simulink model "Quanser_AERO_Simulation_2020b"  (R2020b)
settings: Solver=ode45  StartTime=0.0  StopTime=sim_time  FixedStep=0.01  RelTol=1e-3
InitFcn:
  | % Run simulation parameters
  | quanser_AERO_sim_params;
model workspace (MAT data in the model file):
  a = Simulink.Parameter
  a.Value = 1.15
  a.DataType = 'auto'
  a.Dimensions = [1 1]
  a_a = Simulink.Parameter
  a_a.Value = 0.043381
  a_a.DataType = 'auto'
  a_a.Dimensions = [1 1]
  b = Simulink.Parameter
  b.Value = 0.2847
  b.DataType = 'auto'
  b.Dimensions = [1 1]
  b_b = Simulink.Parameter
  b_b.Value = 0.005
  b_b.DataType = 'auto'
  b_b.Dimensions = [1 1]
  c = Simulink.Parameter
  c.Value = 0.53573
  c.DataType = 'auto'
  c.Dimensions = [1 1]
  c_c = Simulink.Parameter
  c_c.Value = 0.005
  c_c.DataType = 'auto'
  c_c.Dimensions = [1 1]
  d = Simulink.Parameter
  d.Value = 0.0071058
  d.DataType = 'auto'
  d.Dimensions = [1 1]
  d_d = Simulink.Parameter
  d_d.Value = 0
  d_d.DataType = 'auto'
  d_d.Dimensions = [1 1]
  e = Simulink.Parameter
  e.Value = 0.0071
  e.DataType = 'auto'
  e.Dimensions = [1 1]
  f = Simulink.Parameter
  f.Value = 0.05
  f.DataType = 'auto'
  f.Dimensions = [1 1]
  g = Simulink.Parameter
  g.Value = 9.81
  g.DataType = 'auto'
  g.Dimensions = [1 1]
  p_p = Simulink.Parameter
  p_p.Value = 0.0005466
  p_p.DataType = 'auto'
  p_p.Dimensions = [1 1]
  smiData.RigidTransform(1).translation = [75 240 -4.4408920985e-15]
  smiData.RigidTransform(1).angle = 1.57079632679
  smiData.RigidTransform(1).axis = [5.55111512313e-17 1 5.55111512313e-17]
  smiData.RigidTransform(1).ID = 'B[AERO - Fork:1:-:AERO - Arm:1]'
  smiData.RigidTransform(2).translation = [0 0 72.5]
  smiData.RigidTransform(2).angle = 0
  smiData.RigidTransform(2).axis = [0 0 0]
  smiData.RigidTransform(2).ID = 'F[AERO - Fork:1:-:AERO - Arm:1]'
  smiData.RigidTransform(3).translation = [53 0 0]
  smiData.RigidTransform(3).angle = 1.57079632679
  smiData.RigidTransform(3).axis = [0 -1 0]
  smiData.RigidTransform(3).ID = 'B[AERO - Arm:1:-:AERO - Propeller Housing:1]'
  smiData.RigidTransform(4).translation = [-2.67952073108e-14 10 -95.5137103749]
  smiData.RigidTransform(4).angle = 3.14159265359
  smiData.RigidTransform(4).axis = [1 0 0]
  smiData.RigidTransform(4).ID = 'F[AERO - Arm:1:-:AERO - Propeller Housing:1]'
  smiData.RigidTransform(5).translation = [-53 0 0]
  smiData.RigidTransform(5).angle = 3.14159265359
  smiData.RigidTransform(5).axis = [0.707106781187 0 0.707106781187]
  smiData.RigidTransform(5).ID = 'B[AERO - Arm:1:-:AERO - Propeller Housing:2]'
  smiData.RigidTransform(6).translation = [-2.67952073108e-14 10 -95.5137103749]
  smiData.RigidTransform(6).angle = 3.14159265359
  smiData.RigidTransform(6).axis = [1 0 0]
  smiData.RigidTransform(6).ID = 'F[AERO - Arm:1:-:AERO - Propeller Housing:2]'
  smiData.RigidTransform(7).translation = [0 90 0]
  smiData.RigidTransform(7).angle = 2.09439510239
  smiData.RigidTransform(7).axis = [-0.57735026919 -0.57735026919 -0.57735026919]
  smiData.RigidTransform(7).ID = 'B[AERO - Base:1:-:AERO - Fork:1]'
  smiData.RigidTransform(8).translation = [0 -10 -1.83697019872e-15]
  smiData.RigidTransform(8).angle = 1.57079632679
  smiData.RigidTransform(8).axis = [-1 0 0]
  smiData.RigidTransform(8).ID = 'F[AERO - Base:1:-:AERO - Fork:1]'
  smiData.RigidTransform(9).translation = [0 7 0]
  smiData.RigidTransform(9).angle = 1.57079632679
  smiData.RigidTransform(9).axis = [-1 1.5327705937e-16 1.5327705937e-16]
  smiData.RigidTransform(9).ID = 'B[AERO - Propeller Housing:1:-:AERO - Propeller:1]'
  smiData.RigidTransform(10).translation = [0 2 0]
  smiData.RigidTransform(10).angle = 1.6664335536
  smiData.RigidTransform(10).axis = [-0.908660854566 0.295241808844 0.295241808844]
  smiData.RigidTransform(10).ID = 'F[AERO - Propeller Housing:1:-:AERO - Propeller:1]'
  smiData.RigidTransform(11).translation = [0 7 0]
  smiData.RigidTransform(11).angle = 1.57079632679
  smiData.RigidTransform(11).axis = [-1 6.25051204106e-17 6.25051204106e-17]
  smiData.RigidTransform(11).ID = 'B[AERO - Propeller Housing:2:-:AERO - Propeller:2]'
  smiData.RigidTransform(12).translation = [0 2 0]
  smiData.RigidTransform(12).angle = 2.28432867519
  smiData.RigidTransform(12).axis = [-0.456966311669 -0.628960169645 -0.628960169645]
  smiData.RigidTransform(12).ID = 'F[AERO - Propeller Housing:2:-:AERO - Propeller:2]'
  smiData.RigidTransform(13).translation = [-4.21383634609 -51.619496794 8.881784197e-15]
  smiData.RigidTransform(13).angle = 0
  smiData.RigidTransform(13).axis = [0 0 0]
  smiData.RigidTransform(13).ID = 'SixDofRigidTransform[AERO - Base:1]'
  smiData.Solid(1).mass = 2.36460135901
  smiData.Solid(1).CoM = [5.24111117378e-10 37.9532129776 0]
  smiData.Solid(1).MoI = [7187.732483 11870.3385044 7187.73246752]
  smiData.Solid(1).PoI = [0 0 -5.80827271444e-08]
  smiData.Solid(1).color = [0.0196078431373 0.0196078431373 0.0196078431373]
  smiData.Solid(1).opacity = 1
  smiData.Solid(1).ID = 'AERO - Base.ipt_{5B170AF7-4835-771C-6ADF-04BDBD784493}'
  smiData.Solid(2).mass = 0.833057949362
  smiData.Solid(2).CoM = [2.66169728603e-11 94.8876622043 1.47659785864e-12]
  smiData.Solid(2).MoI = [5303.1260885 5291.93963258 10383.1205417]
  smiData.Solid(2).PoI = [-1.78319566538e-10 1.20053300634e-10 2.21603950608e-09]
  smiData.Solid(2).color = [0.0196078431373 0.0196078431373 0.0196078431373]
  smiData.Solid(2).opacity = 1
  smiData.Solid(2).ID = 'AERO - Fork.ipt_{19DEB560-4DA8-F02E-E9C0-369FCF880C44}'
  smiData.Solid(3).mass = 0.268036846773
  smiData.Solid(3).CoM = [1.42171296006e-09 -5.19659809406e-10 0]
  smiData.Solid(3).MoI = [365.292105474 461.18513674 151.85502279]
  smiData.Solid(3).PoI = [9.09494701773e-14 -7.58518581279e-10 0]
  smiData.Solid(3).color = [0.0196078431373 0.0196078431373 0.0196078431373]
  smiData.Solid(3).opacity = 1
  smiData.Solid(3).ID = 'AERO - Arm.ipt_{15B1D815-460D-A329-2F9F-5FB9E93ED37B}'
  smiData.Solid(4).mass = 0.12383177107
  smiData.Solid(4).CoM = [0.00177195297055 5.45503898669 -8.60877968745]
  smiData.Solid(4).MoI = [310.701431452 411.715449483 138.600608927]
  smiData.Solid(4).PoI = [4.84491065682 -0.146839869659 -0.00100363322073]
  smiData.Solid(4).color = [0.0196078431373 0.0196078431373 0.0196078431373]
  smiData.Solid(4).opacity = 1
  smiData.Solid(4).ID = 'AERO - Propeller Housing.ipt_{180F9119-4C93-59E3-A88D-3BA97F46F3C3}'
  smiData.Solid(5).mass = 0.0206425497221
  smiData.Solid(5).CoM = [-1.0654070865e-12 5.09575570658 -2.10819251568e-11]
  smiData.Solid(5).MoI = [13.8216638961 27.2772869122 13.8216638974]
  smiData.Solid(5).PoI = [0 0 -9.39933149128e-14]
  smiData.Solid(5).color = [0.121568627451 0.121568627451 0.705882352941]
  smiData.Solid(5).opacity = 1
  smiData.Solid(5).ID = 'AERO - Propeller.ipt_{54ECD9B7-47A0-F6BB-CE8E-F5BB4731363E}'
  smiData.RevoluteJoint(1).Rz.Pos = 8.54433050095e-10
  smiData.RevoluteJoint(1).ID = '[AERO - Fork:1:-:AERO - Arm:1]'
  smiData.RevoluteJoint(2).Rz.Pos = 176.894023419
  smiData.RevoluteJoint(2).ID = '[AERO - Arm:1:-:AERO - Propeller Housing:1]'
  smiData.RevoluteJoint(3).Rz.Pos = 3.10597658118
  smiData.RevoluteJoint(3).ID = '[AERO - Arm:1:-:AERO - Propeller Housing:2]'
  smiData.RevoluteJoint(4).Rz.Pos = -4.73234748156e-11
  smiData.RevoluteJoint(4).ID = '[AERO - Base:1:-:AERO - Fork:1]'
  smiData.RevoluteJoint(5).Rz.Pos = -5.89066785065e-05
  smiData.RevoluteJoint(5).ID = '[AERO - Propeller Housing:1:-:AERO - Propeller:1]'
  smiData.RevoluteJoint(6).Rz.Pos = -3.64250166753e-05
  smiData.RevoluteJoint(6).ID = '[AERO - Propeller Housing:2:-:AERO - Propeller:2]'
  t_t = Simulink.Parameter
  t_t.Value = 0.0005466
  t_t.DataType = 'auto'
  t_t.Dimensions = [1 1]
  u_lim = Simulink.Parameter
  u_lim.Value = 24
  u_lim.DataType = 'auto'
  u_lim.Dimensions = [1 1]
  y_y = Simulink.Parameter
  y_y.Value = 0.02
  y_y.DataType = 'auto'
  y_y.Dimensions = [1 1]
  z_z = Simulink.Parameter
  z_z.Value = 0.01
  z_z.DataType = 'auto'
  z_z.Dimensions = [1 1]
undefined symbols (not defined in the file): ini_cond, K_cr, K_D, K_I, K_P, model, noise, tau_p, ts, X, Y, Z
libraries: sm_lib x140, nesl_utility x28, simulink x24
(part 1 of 4)
settings Model: DataDictionary=AERO_DigitalTwin.sldd  OrderedModelArguments=off  Creator=garciar1  LastModifiedBy=linesLK
settings ExplorerConfigSet: InternalSimMechanicsExplorerSettings="<ExplorerConfiguration><canonicalview>planar_xy</canonicalview><AnimationSetting><BasePlaybackSpeed>1.0</BasePlaybackSpeed><PlaybackSpeedFactor>1.0</PlaybackSpeedFactor></AnimationSetting><TilePanel><TileInfo><Tiles Columns=\"1\" Count=\"1\" Rows=\"1\"><Column Weight=\"1\"/><Row Weight=\"1\"/><Tile Height=\"1\" Width=\"1\" X=\"0\" Y=\"0\"/></Tiles></TileInfo><SceneInfo><SceneViewer><BGColor><R>0.60000002384185791</R><G>0.60000002384185791</G><B>0.60000002384185791</B></BGColor><Camera><DoPerspective>off</DoPerspective><Position><X>0.606138610969192748</X><Y>0.738169372517540556</Y><Z>0.590514966088055981</Z></Position><Center><X>0.0287883417795668992</X><Y>0.160819103327914742</Y><Z>0.0131646968984300838</Z></Center><Up><X>-0.408248290463863073</X><Y>0.816496580927726145</Y><Z>-0.408248290463863073</Z></Up><ViewLimDist>1</ViewLimDist><YLim>0.238299283981323246</YLim><XLim>0.228027763120059318</XLim></Camera></SceneViewer></SceneInfo></TilePanel><MechEditorPanel><Cameras/><GfxPanelCameraMap/><VideoCreator><PlaybackSpeedRatio>1.0</PlaybackSpeedRatio><FrameRate>30</FrameRate><VideoFormat>Motion JPEG AVI</VideoFormat><FrameSize>auto</FrameSize></VideoCreator></MechEditorPanel></ExplorerConfiguration>"

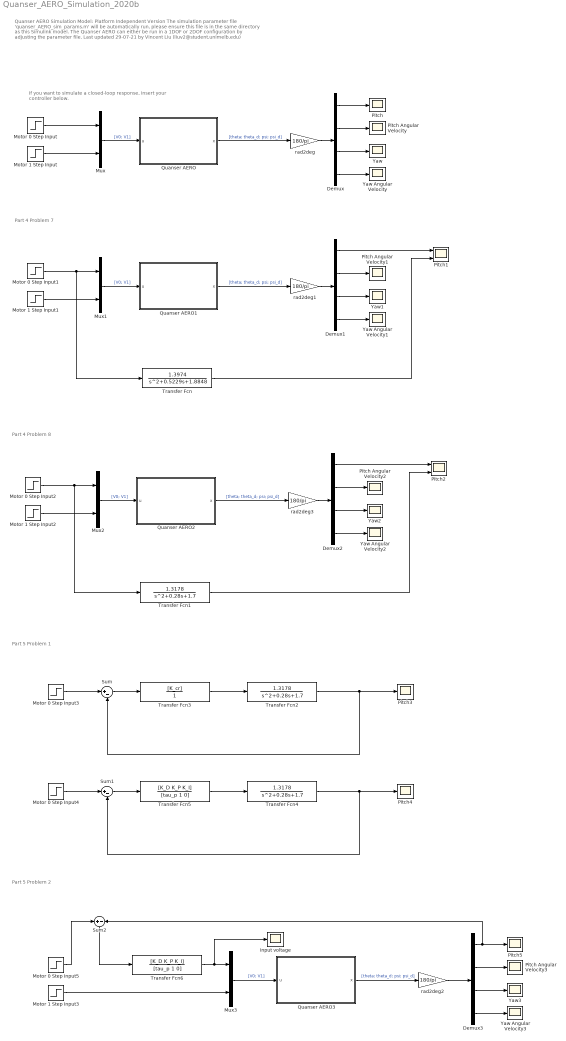
== system Quanser_AERO_Simulation_2020b ==
  note: If you want to simulate a closed-loop response, insert your controller below.
  note: Quanser AERO Simulation Model: Platform Independent Version
      | The simulation parameter file 'quanser_AERO_sim_params.m' will be automatically run, please ensure this file is in the same directory as this Simulink model. The Quanser AERO can either be run in a 1DOF or 2DOF configuration by adjusting the parameter file.
      | Last updated 29-07-21 by Vincent Liu (liuv2@student.unimelb.edu)
  note: Part 4 Problem 7
  note: Part 4 Problem 8
  note: Part 5 Problem 1
  note: Part 5 Problem 2
  Demux{,1..3} (4 alike) : Demux
  Motor 0 Step Input{,1..4} (5 alike) : Step  After=20  SampleTime=0
  Motor 0 Step Input5 : Step  After=10  SampleTime=0
  Motor 1 Step Input{,1..3} (4 alike) : Step  After=10  SampleTime=0
  Mux{,1..3} (4 alike) : Mux  Inputs=2
  Pitch{,3..5} (4 alike) : Scope
  Pitch Angular Velocity{,1..3} (4 alike) : Scope
  Pitch1 : Scope  NumInputPorts=2
  Pitch2 : Scope  NumInputPorts=2
  Quanser AERO : Subsystem  TreatAsAtomicUnit=on
  Quanser AERO1 : Subsystem  TreatAsAtomicUnit=on
  Quanser AERO2 : Subsystem  TreatAsAtomicUnit=on
  Quanser AERO3 : Subsystem  TreatAsAtomicUnit=on
  Sum : Sum  Inputs=|+-
  Sum1 : Sum  Inputs=|+-
  Sum2 : Sum  Inputs=+-
  Transfer Fcn : TransferFcn  Numerator=[1.3974]  Denominator=[1 0.5229 1.8848]
  Transfer Fcn1 : TransferFcn  Numerator=[1.3178]  Denominator=[1 0.28 1.7]
  Transfer Fcn2 : TransferFcn  Numerator=[1.3178]  Denominator=[1 0.28 1.7]
  Transfer Fcn3 : TransferFcn  Numerator=[K_cr]  Denominator=1
  Transfer Fcn4 : TransferFcn  Numerator=[1.3178]  Denominator=[1 0.28 1.7]
  Transfer Fcn5 : TransferFcn  Numerator=[K_D K_P K_I]  Denominator=[tau_p 1 0]
  Transfer Fcn6 : TransferFcn  Numerator=[K_D K_P K_I]  Denominator=[tau_p 1 0]
  Yaw{,1..3} (4 alike) : Scope
  Yaw Angular Velocity{,1..3} (4 alike) : Scope
  input voltage : Scope
  rad2deg{,1..3} (4 alike) : Gain  Gain=180/pi
  wires:
  Demux/3 -> Yaw/1
  Demux/2 -> Pitch Angular Velocity/1
  Demux/4 -> Yaw Angular Velocity/1
  Mux/1 -> Quanser AERO/1(u)  "[V0; V1]"
  rad2deg/1 -> Demux/1
  Quanser AERO/1(x) -> rad2deg/1  "[theta; theta_d; psi; psi_d]"
  Motor 1 Step Input/1 -> Mux/2
  Motor 0 Step Input/1 -> Mux/1
  Demux/1 -> Pitch/1
  Demux1/4 -> Yaw Angular Velocity1/1
  rad2deg1/1 -> Demux1/1
  Demux1/3 -> Yaw1/1
  Quanser AERO1/1(x) -> rad2deg1/1  "[theta; theta_d; psi; psi_d]"
  Mux1/1 -> Quanser AERO1/1(u)  "[V0; V1]"
  Motor 1 Step Input1/1 -> Mux1/2
  Motor 0 Step Input1/1 -> Transfer Fcn/1, Mux1/1
  Demux1/2 -> Pitch Angular Velocity1/1
  Demux1/1 -> Pitch1/1
  Transfer Fcn/1 -> Pitch1/2
  Demux2/3 -> Yaw2/1
  Demux2/4 -> Yaw Angular Velocity2/1
  Demux2/1 -> Pitch2/1
  rad2deg3/1 -> Demux2/1
  Quanser AERO2/1(x) -> rad2deg3/1  "[theta; theta_d; psi; psi_d]"
  Mux2/1 -> Quanser AERO2/1(u)  "[V0; V1]"
  Demux2/2 -> Pitch Angular Velocity2/1
  Transfer Fcn1/1 -> Pitch2/2
  Motor 1 Step Input2/1 -> Mux2/2
  Motor 0 Step Input2/1 -> Transfer Fcn1/1, Mux2/1
  Transfer Fcn2/1 -> Pitch3/1, Sum/2
  Transfer Fcn3/1 -> Transfer Fcn2/1
  Motor 0 Step Input3/1 -> Sum/1
  Sum/1 -> Transfer Fcn3/1
  Transfer Fcn5/1 -> Transfer Fcn4/1
  Transfer Fcn4/1 -> Sum1/2, Pitch4/1
  Sum1/1 -> Transfer Fcn5/1
  Motor 0 Step Input4/1 -> Sum1/1
  rad2deg2/1 -> Demux3/1
  Demux3/1 -> Pitch5/1, Sum2/2
  Demux3/4 -> Yaw Angular Velocity3/1
  Demux3/3 -> Yaw3/1
  Demux3/2 -> Pitch Angular Velocity3/1
  Motor 1 Step Input3/1 -> Mux3/2
  Quanser AERO3/1(x) -> rad2deg2/1  "[theta; theta_d; psi; psi_d]"
  Mux3/1 -> Quanser AERO3/1(u)  "[V0; V1]"
  Transfer Fcn6/1 -> input voltage/1, Mux3/1
  Motor 0 Step Input5/1 -> Sum2/1
  Sum2/1 -> Transfer Fcn6/1

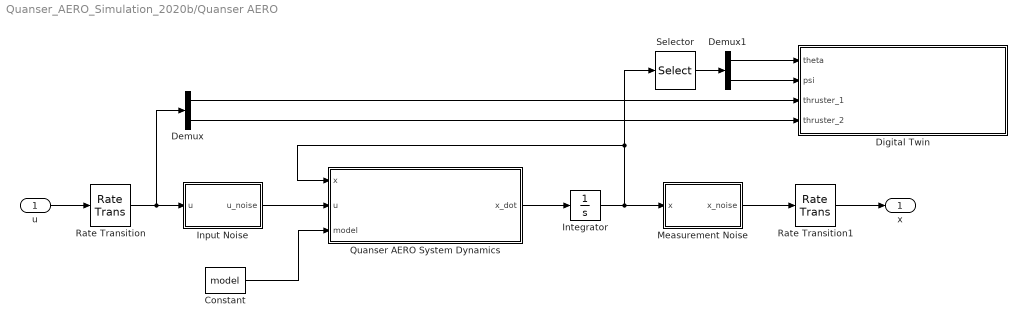
== system Quanser_AERO_Simulation_2020b/Quanser AERO ==
  u : Inport
  Constant : Constant  Value=model
  Demux : Demux  Outputs=2
  Demux1 : Demux  Outputs=2
  Digital Twin : Subsystem
  Input Noise : Subsystem  TreatAsAtomicUnit=on
  Integrator : Integrator  InitialCondition=[ini_cond.theta; ini_cond.theta_dot; ini_cond.psi; ini_cond.psi_dot]
  Measurement Noise : Subsystem  TreatAsAtomicUnit=on
  Quanser AERO System Dynamics : Subsystem  TreatAsAtomicUnit=on
  Rate Transition : RateTransition  OutPortSampleTime=ts
  Rate Transition1 : RateTransition  InitialCondition=[ini_cond.theta; ini_cond.theta_dot; ini_cond.psi; ini_cond.psi_dot]  OutPortSampleTime=ts
  Selector : Selector  InputPortWidth=4  IndexOptions=Index vector (dialog)  Indices=[1 3]  OutputSizes=1
  x : Outport  VectorParamsAs1DForOutWhenUnconnected=off
  wires:
  u/1 -> Rate Transition/1
  Rate Transition/1 -> Input Noise/1(u), Demux/1
  Rate Transition1/1 -> x/1
  Input Noise/1(u_noise) -> Quanser AERO System Dynamics/2(u)
  Measurement Noise/1(x_noise) -> Rate Transition1/1
  Selector/1 -> Demux1/1
  Demux/1 -> Digital Twin/3(thruster_1)
  Demux/2 -> Digital Twin/4(thruster_2)
  Demux1/1 -> Digital Twin/1(theta)
  Demux1/2 -> Digital Twin/2(psi)
  Integrator/1 -> Measurement Noise/1(x), Selector/1, Quanser AERO System Dynamics/1(x)
  Constant/1 -> Quanser AERO System Dynamics/3(model)
  Quanser AERO System Dynamics/1(x_dot) -> Integrator/1

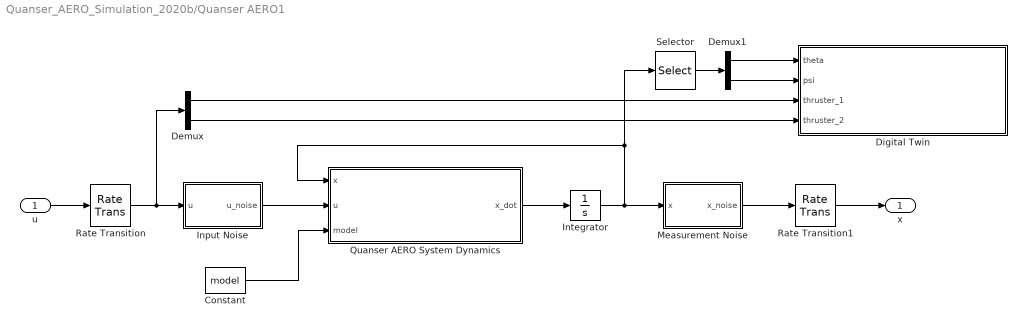
== system Quanser_AERO_Simulation_2020b/Quanser AERO1 ==
  u : Inport
  Constant : Constant  Value=model
  Demux : Demux  Outputs=2
  Demux1 : Demux  Outputs=2
  Digital Twin : Subsystem
  Input Noise : Subsystem  TreatAsAtomicUnit=on
  Integrator : Integrator  InitialCondition=[ini_cond.theta; ini_cond.theta_dot; ini_cond.psi; ini_cond.psi_dot]
  Measurement Noise : Subsystem  TreatAsAtomicUnit=on
  Quanser AERO System Dynamics : Subsystem  TreatAsAtomicUnit=on
  Rate Transition : RateTransition  OutPortSampleTime=ts
  Rate Transition1 : RateTransition  InitialCondition=[ini_cond.theta; ini_cond.theta_dot; ini_cond.psi; ini_cond.psi_dot]  OutPortSampleTime=ts
  Selector : Selector  InputPortWidth=4  IndexOptions=Index vector (dialog)  Indices=[1 3]  OutputSizes=1
  x : Outport  VectorParamsAs1DForOutWhenUnconnected=off
  wires:
  u/1 -> Rate Transition/1
  Rate Transition/1 -> Input Noise/1(u), Demux/1
  Rate Transition1/1 -> x/1
  Input Noise/1(u_noise) -> Quanser AERO System Dynamics/2(u)
  Measurement Noise/1(x_noise) -> Rate Transition1/1
  Selector/1 -> Demux1/1
  Demux/1 -> Digital Twin/3(thruster_1)
  Demux/2 -> Digital Twin/4(thruster_2)
  Demux1/1 -> Digital Twin/1(theta)
  Demux1/2 -> Digital Twin/2(psi)
  Integrator/1 -> Measurement Noise/1(x), Selector/1, Quanser AERO System Dynamics/1(x)
  Constant/1 -> Quanser AERO System Dynamics/3(model)
  Quanser AERO System Dynamics/1(x_dot) -> Integrator/1

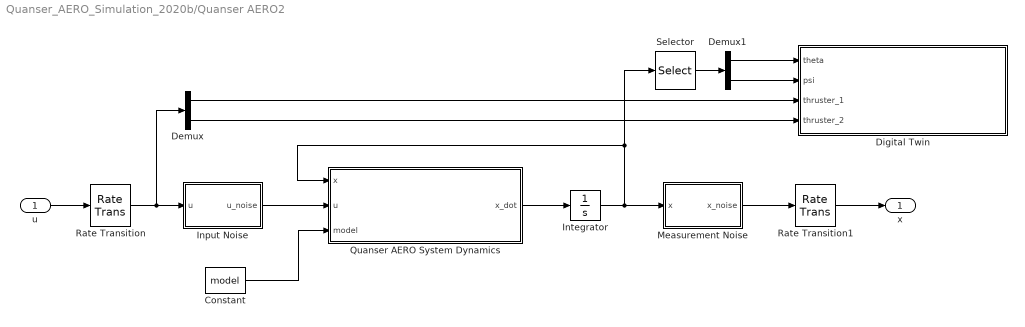
== system Quanser_AERO_Simulation_2020b/Quanser AERO2 ==
  u : Inport
  Constant : Constant  Value=model
  Demux : Demux  Outputs=2
  Demux1 : Demux  Outputs=2
  Digital Twin : Subsystem
  Input Noise : Subsystem  TreatAsAtomicUnit=on
  Integrator : Integrator  InitialCondition=[ini_cond.theta; ini_cond.theta_dot; ini_cond.psi; ini_cond.psi_dot]
  Measurement Noise : Subsystem  TreatAsAtomicUnit=on
  Quanser AERO System Dynamics : Subsystem  TreatAsAtomicUnit=on
  Rate Transition : RateTransition  OutPortSampleTime=ts
  Rate Transition1 : RateTransition  InitialCondition=[ini_cond.theta; ini_cond.theta_dot; ini_cond.psi; ini_cond.psi_dot]  OutPortSampleTime=ts
  Selector : Selector  InputPortWidth=4  IndexOptions=Index vector (dialog)  Indices=[1 3]  OutputSizes=1
  x : Outport  VectorParamsAs1DForOutWhenUnconnected=off
  wires:
  u/1 -> Rate Transition/1
  Rate Transition/1 -> Input Noise/1(u), Demux/1
  Rate Transition1/1 -> x/1
  Input Noise/1(u_noise) -> Quanser AERO System Dynamics/2(u)
  Measurement Noise/1(x_noise) -> Rate Transition1/1
  Selector/1 -> Demux1/1
  Demux/1 -> Digital Twin/3(thruster_1)
  Demux/2 -> Digital Twin/4(thruster_2)
  Demux1/1 -> Digital Twin/1(theta)
  Demux1/2 -> Digital Twin/2(psi)
  Integrator/1 -> Measurement Noise/1(x), Selector/1, Quanser AERO System Dynamics/1(x)
  Constant/1 -> Quanser AERO System Dynamics/3(model)
  Quanser AERO System Dynamics/1(x_dot) -> Integrator/1

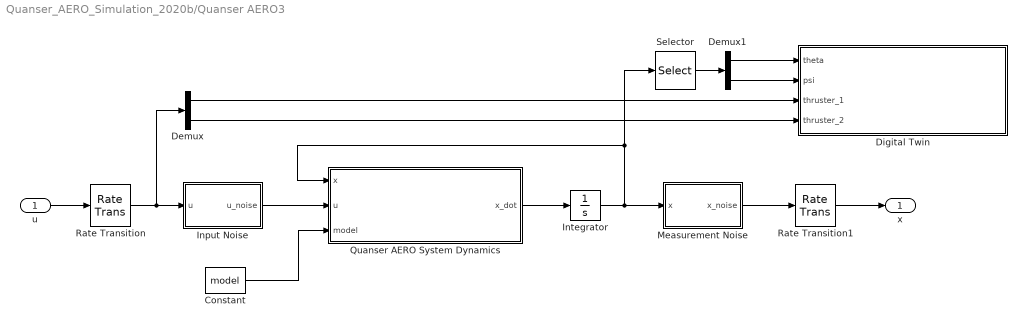
== system Quanser_AERO_Simulation_2020b/Quanser AERO3 ==
  u : Inport
  Constant : Constant  Value=model
  Demux : Demux  Outputs=2
  Demux1 : Demux  Outputs=2
  Digital Twin : Subsystem
  Input Noise : Subsystem  TreatAsAtomicUnit=on
  Integrator : Integrator  InitialCondition=[ini_cond.theta; ini_cond.theta_dot; ini_cond.psi; ini_cond.psi_dot]
  Measurement Noise : Subsystem  TreatAsAtomicUnit=on
  Quanser AERO System Dynamics : Subsystem  TreatAsAtomicUnit=on
  Rate Transition : RateTransition  OutPortSampleTime=ts
  Rate Transition1 : RateTransition  InitialCondition=[ini_cond.theta; ini_cond.theta_dot; ini_cond.psi; ini_cond.psi_dot]  OutPortSampleTime=ts
  Selector : Selector  InputPortWidth=4  IndexOptions=Index vector (dialog)  Indices=[1 3]  OutputSizes=1
  x : Outport  VectorParamsAs1DForOutWhenUnconnected=off
  wires:
  u/1 -> Rate Transition/1
  Rate Transition/1 -> Input Noise/1(u), Demux/1
  Rate Transition1/1 -> x/1
  Input Noise/1(u_noise) -> Quanser AERO System Dynamics/2(u)
  Measurement Noise/1(x_noise) -> Rate Transition1/1
  Selector/1 -> Demux1/1
  Demux/1 -> Digital Twin/3(thruster_1)
  Demux/2 -> Digital Twin/4(thruster_2)
  Demux1/1 -> Digital Twin/1(theta)
  Demux1/2 -> Digital Twin/2(psi)
  Integrator/1 -> Measurement Noise/1(x), Selector/1, Quanser AERO System Dynamics/1(x)
  Constant/1 -> Quanser AERO System Dynamics/3(model)
  Quanser AERO System Dynamics/1(x_dot) -> Integrator/1

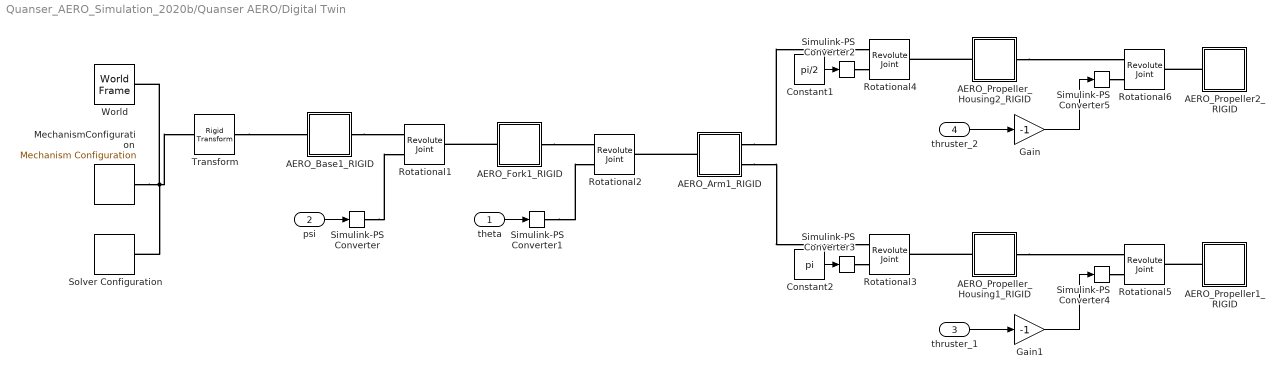
== system Quanser_AERO_Simulation_2020b/Quanser AERO/Digital Twin ==
  theta : Inport
  psi : Inport  Port=2
  thruster_1 : Inport  Port=3
  thruster_2 : Inport  Port=4
  AERO_Arm1_RIGID : Subsystem
  AERO_Base1_RIGID : Subsystem
  AERO_Fork1_RIGID : Subsystem
  AERO_Propeller1_RIGID : Subsystem
  AERO_Propeller2_RIGID : Subsystem
  AERO_Propeller_Housing1_RIGID : Subsystem
  AERO_Propeller_Housing2_RIGID : Subsystem
  Constant1 : Constant  Value=pi/2
  Constant2 : Constant  Value=pi
  Gain : Gain  Gain=-1
  Gain1 : Gain  Gain=-1
  MechanismConfiguration : sm_lib/Utilities/Mechanism Configuration  UniformGravity=Constant  GravityVector=[0 -9.80665 0]  GravityVectorUnits=m/s^2  GravityUnits=m/s^2  LinearizationDelta=0.001  JointModeTransitionNonlinearIterations=2
  Rotational1 : sm_lib/Joints/Revolute Joint  JointMode=Normal  SenseConstraintForce=off  SenseConstraintForceX=off  SenseConstraintForceY=off  SenseConstraintForceZ=off  SenseConstraintTorque=off  SenseConstraintTorqueX=off  SenseConstraintTorqueY=off  SenseConstraintTorqueZ=off  SenseTotalForce=off  SenseTotalForceX=off  SenseTotalForceY=off  SenseTotalForceZ=off  SenseTotalTorque=off  SenseTotalTorqueX=off  SenseTotalTorqueY=off  SenseTotalTorqueZ=off  CompositeWrenchDir=FollowerOnBase  CompositeWrenchFrame=BaseFrame  EquilibriumPosition=0  EquilibriumPositionUnits=deg  SpringStiffness=0  SpringStiffnessUnits=N*m/deg  DampingCoefficient=0  DampingCoefficientUnits=N*m/(deg/s)  TorqueActuationMode=ComputedTorque  MotionActuationMode=InputMotion  SensePosition=off  SenseVelocity=off  SenseAcceleration=off  SenseTorqueForce=off  SenseLowerLimitTorqueForce=off  SenseUpperLimitTorqueForce=off  LowerLimitSpecify=off  LowerLimitBound=-90  LowerLimitBoundUnits=deg  LowerLimitStiffness=1e4  LowerLimitStiffnessUnits=N*m/deg  LowerLimitDamping=10  LowerLimitDampingUnits=N*m/(deg/s)  LowerLimitTransitionRegionWidth=0.1  LowerLimitTransitionRegionWidthUnits=deg  UpperLimitSpecify=off  UpperLimitBound=90  UpperLimitBoundUnits=deg  UpperLimitStiffness=1e4  UpperLimitStiffnessUnits=N*m/deg  UpperLimitDamping=10  UpperLimitDampingUnits=N*m/(deg/s)  UpperLimitTransitionRegionWidth=0.1  UpperLimitTransitionRegionWidthUnits=deg  PositionTargetSpecify=on  PositionTargetPriority=Low  PositionTargetValue=smiData.RevoluteJoint(4).Rz.Pos  PositionTargetValueUnits=deg  VelocityTargetSpecify=off  VelocityTargetPriority=High  VelocityTargetValue=0  VelocityTargetValueUnits=deg/s
  Rotational2 : sm_lib/Joints/Revolute Joint  JointMode=Normal  SenseConstraintForce=off  SenseConstraintForceX=off  SenseConstraintForceY=off  SenseConstraintForceZ=off  SenseConstraintTorque=off  SenseConstraintTorqueX=off  SenseConstraintTorqueY=off  SenseConstraintTorqueZ=off  SenseTotalForce=off  SenseTotalForceX=off  SenseTotalForceY=off  SenseTotalForceZ=off  SenseTotalTorque=off  SenseTotalTorqueX=off  SenseTotalTorqueY=off  SenseTotalTorqueZ=off  CompositeWrenchDir=FollowerOnBase  CompositeWrenchFrame=BaseFrame  EquilibriumPosition=0  EquilibriumPositionUnits=deg  SpringStiffness=0  SpringStiffnessUnits=N*m/deg  DampingCoefficient=0  DampingCoefficientUnits=N*m/(deg/s)  TorqueActuationMode=ComputedTorque  MotionActuationMode=InputMotion  SensePosition=off  SenseVelocity=off  SenseAcceleration=off  SenseTorqueForce=off  SenseLowerLimitTorqueForce=off  SenseUpperLimitTorqueForce=off  LowerLimitSpecify=off  LowerLimitBound=-90  LowerLimitBoundUnits=deg  LowerLimitStiffness=1e4  LowerLimitStiffnessUnits=N*m/deg  LowerLimitDamping=10  LowerLimitDampingUnits=N*m/(deg/s)  LowerLimitTransitionRegionWidth=0.1  LowerLimitTransitionRegionWidthUnits=deg  UpperLimitSpecify=off  UpperLimitBound=90  UpperLimitBoundUnits=deg  UpperLimitStiffness=1e4  UpperLimitStiffnessUnits=N*m/deg  UpperLimitDamping=10  UpperLimitDampingUnits=N*m/(deg/s)  UpperLimitTransitionRegionWidth=0.1  UpperLimitTransitionRegionWidthUnits=deg  PositionTargetSpecify=on  PositionTargetPriority=Low  PositionTargetValue=smiData.RevoluteJoint(1).Rz.Pos  PositionTargetValueUnits=deg  VelocityTargetSpecify=off  VelocityTargetPriority=High  VelocityTargetValue=0  VelocityTargetValueUnits=deg/s
  Rotational3 : sm_lib/Joints/Revolute Joint  JointMode=Normal  SenseConstraintForce=off  SenseConstraintForceX=off  SenseConstraintForceY=off  SenseConstraintForceZ=off  SenseConstraintTorque=off  SenseConstraintTorqueX=off  SenseConstraintTorqueY=off  SenseConstraintTorqueZ=off  SenseTotalForce=off  SenseTotalForceX=off  SenseTotalForceY=off  SenseTotalForceZ=off  SenseTotalTorque=off  SenseTotalTorqueX=off  SenseTotalTorqueY=off  SenseTotalTorqueZ=off  CompositeWrenchDir=FollowerOnBase  CompositeWrenchFrame=BaseFrame  EquilibriumPosition=0  EquilibriumPositionUnits=deg  SpringStiffness=0  SpringStiffnessUnits=N*m/deg  DampingCoefficient=0  DampingCoefficientUnits=N*m/(deg/s)  TorqueActuationMode=ComputedTorque  MotionActuationMode=InputMotion  SensePosition=off  SenseVelocity=off  SenseAcceleration=off  SenseTorqueForce=off  SenseLowerLimitTorqueForce=off  SenseUpperLimitTorqueForce=off  LowerLimitSpecify=off  LowerLimitBound=-90  LowerLimitBoundUnits=deg  LowerLimitStiffness=1e4  LowerLimitStiffnessUnits=N*m/deg  LowerLimitDamping=10  LowerLimitDampingUnits=N*m/(deg/s)  LowerLimitTransitionRegionWidth=0.1  LowerLimitTransitionRegionWidthUnits=deg  UpperLimitSpecify=off  UpperLimitBound=90  UpperLimitBoundUnits=deg  UpperLimitStiffness=1e4  UpperLimitStiffnessUnits=N*m/deg  UpperLimitDamping=10  UpperLimitDampingUnits=N*m/(deg/s)  UpperLimitTransitionRegionWidth=0.1  UpperLimitTransitionRegionWidthUnits=deg  PositionTargetSpecify=on  PositionTargetPriority=High  PositionTargetValue=smiData.RevoluteJoint(2).Rz.Pos  PositionTargetValueUnits=deg  VelocityTargetSpecify=off  VelocityTargetPriority=High  VelocityTargetValue=0  VelocityTargetValueUnits=deg/s
  Rotational4 : sm_lib/Joints/Revolute Joint  JointMode=Normal  SenseConstraintForce=off  SenseConstraintForceX=off  SenseConstraintForceY=off  SenseConstraintForceZ=off  SenseConstraintTorque=off  SenseConstraintTorqueX=off  SenseConstraintTorqueY=off  SenseConstraintTorqueZ=off  SenseTotalForce=off  SenseTotalForceX=off  SenseTotalForceY=off  SenseTotalForceZ=off  SenseTotalTorque=off  SenseTotalTorqueX=off  SenseTotalTorqueY=off  SenseTotalTorqueZ=off  CompositeWrenchDir=FollowerOnBase  CompositeWrenchFrame=BaseFrame  EquilibriumPosition=0  EquilibriumPositionUnits=deg  SpringStiffness=0  SpringStiffnessUnits=N*m/deg  DampingCoefficient=0  DampingCoefficientUnits=N*m/(deg/s)  TorqueActuationMode=ComputedTorque  MotionActuationMode=InputMotion  SensePosition=off  SenseVelocity=off  SenseAcceleration=off  SenseTorqueForce=off  SenseLowerLimitTorqueForce=off  SenseUpperLimitTorqueForce=off  LowerLimitSpecify=off  LowerLimitBound=-90  LowerLimitBoundUnits=deg  LowerLimitStiffness=1e4  LowerLimitStiffnessUnits=N*m/deg  LowerLimitDamping=10  LowerLimitDampingUnits=N*m/(deg/s)  LowerLimitTransitionRegionWidth=0.1  LowerLimitTransitionRegionWidthUnits=deg  UpperLimitSpecify=off  UpperLimitBound=90  UpperLimitBoundUnits=deg  UpperLimitStiffness=1e4  UpperLimitStiffnessUnits=N*m/deg  UpperLimitDamping=10  UpperLimitDampingUnits=N*m/(deg/s)  UpperLimitTransitionRegionWidth=0.1  UpperLimitTransitionRegionWidthUnits=deg  PositionTargetSpecify=on  PositionTargetPriority=Low  PositionTargetValue=smiData.RevoluteJoint(3).Rz.Pos  PositionTargetValueUnits=deg  VelocityTargetSpecify=off  VelocityTargetPriority=High  VelocityTargetValue=0  VelocityTargetValueUnits=deg/s
  Rotational5 : sm_lib/Joints/Revolute Joint  JointMode=Normal  SenseConstraintForce=off  SenseConstraintForceX=off  SenseConstraintForceY=off  SenseConstraintForceZ=off  SenseConstraintTorque=off  SenseConstraintTorqueX=off  SenseConstraintTorqueY=off  SenseConstraintTorqueZ=off  SenseTotalForce=off  SenseTotalForceX=off  SenseTotalForceY=off  SenseTotalForceZ=off  SenseTotalTorque=off  SenseTotalTorqueX=off  SenseTotalTorqueY=off  SenseTotalTorqueZ=off  CompositeWrenchDir=FollowerOnBase  CompositeWrenchFrame=BaseFrame  EquilibriumPosition=0  EquilibriumPositionUnits=deg  SpringStiffness=0  SpringStiffnessUnits=N*m/deg  DampingCoefficient=0.000001  DampingCoefficientUnits=N*m/(deg/s)  TorqueActuationMode=InputTorque  MotionActuationMode=ComputedMotion  SensePosition=off  SenseVelocity=off  SenseAcceleration=off  SenseTorqueForce=off  SenseLowerLimitTorqueForce=off  SenseUpperLimitTorqueForce=off  LowerLimitSpecify=off  LowerLimitBound=-90  LowerLimitBoundUnits=deg  LowerLimitStiffness=1e4  LowerLimitStiffnessUnits=N*m/deg  LowerLimitDamping=10  LowerLimitDampingUnits=N*m/(deg/s)  LowerLimitTransitionRegionWidth=0.1  LowerLimitTransitionRegionWidthUnits=deg  UpperLimitSpecify=off  UpperLimitBound=90  UpperLimitBoundUnits=deg  UpperLimitStiffness=1e4  UpperLimitStiffnessUnits=N*m/deg  UpperLimitDamping=10  UpperLimitDampingUnits=N*m/(deg/s)  UpperLimitTransitionRegionWidth=0.1  UpperLimitTransitionRegionWidthUnits=deg  PositionTargetSpecify=on  PositionTargetPriority=Low  PositionTargetValue=smiData.RevoluteJoint(5).Rz.Pos  PositionTargetValueUnits=deg  VelocityTargetSpecify=off  VelocityTargetPriority=High  VelocityTargetValue=0  VelocityTargetValueUnits=deg/s
  Rotational6 : sm_lib/Joints/Revolute Joint  JointMode=Normal  SenseConstraintForce=off  SenseConstraintForceX=off  SenseConstraintForceY=off  SenseConstraintForceZ=off  SenseConstraintTorque=off  SenseConstraintTorqueX=off  SenseConstraintTorqueY=off  SenseConstraintTorqueZ=off  SenseTotalForce=off  SenseTotalForceX=off  SenseTotalForceY=off  SenseTotalForceZ=off  SenseTotalTorque=off  SenseTotalTorqueX=off  SenseTotalTorqueY=off  SenseTotalTorqueZ=off  CompositeWrenchDir=FollowerOnBase  CompositeWrenchFrame=BaseFrame  EquilibriumPosition=0  EquilibriumPositionUnits=deg  SpringStiffness=0  SpringStiffnessUnits=N*m/deg  DampingCoefficient=0.000001  DampingCoefficientUnits=N*m/(rad/s)  TorqueActuationMode=InputTorque  MotionActuationMode=ComputedMotion  SensePosition=off  SenseVelocity=off  SenseAcceleration=off  SenseTorqueForce=off  SenseLowerLimitTorqueForce=off  SenseUpperLimitTorqueForce=off  LowerLimitSpecify=off  LowerLimitBound=-90  LowerLimitBoundUnits=deg  LowerLimitStiffness=1e4  LowerLimitStiffnessUnits=N*m/deg  LowerLimitDamping=10  LowerLimitDampingUnits=N*m/(deg/s)  LowerLimitTransitionRegionWidth=0.1  LowerLimitTransitionRegionWidthUnits=deg  UpperLimitSpecify=off  UpperLimitBound=90  UpperLimitBoundUnits=deg  UpperLimitStiffness=1e4  UpperLimitStiffnessUnits=N*m/deg  UpperLimitDamping=10  UpperLimitDampingUnits=N*m/(deg/s)  UpperLimitTransitionRegionWidth=0.1  UpperLimitTransitionRegionWidthUnits=deg  PositionTargetSpecify=on  PositionTargetPriority=Low  PositionTargetValue=smiData.RevoluteJoint(6).Rz.Pos  PositionTargetValueUnits=deg  VelocityTargetSpecify=off  VelocityTargetPriority=High  VelocityTargetValue=0  VelocityTargetValueUnits=deg/s
  Simulink-PS Converter{,1..3} (4 alike) : nesl_utility/Simulink-PS Converter  PhysicalDomain=network_engine_domain  SubClassName=ps_input  LeftPortType=input  RightPortType=output  PseudoPeriodic=off  Frequencies=[]  NoiseDistribution=none  NoiseParameters=[]  Unit=1  AffineConversion=off  FilteringAndDerivatives=filter  SimscapeFilterOrder=2  InputFilterTimeConstant=0.001  UdotUserProvided=0
      settings: SourceProductBaseCode=PW,SS
  Simulink-PS Converter4 : nesl_utility/Simulink-PS Converter  PhysicalDomain=network_engine_domain  SubClassName=ps_input  LeftPortType=input  RightPortType=output  PseudoPeriodic=off  Frequencies=[]  NoiseDistribution=none  NoiseParameters=[]  Unit=1  AffineConversion=off  FilteringAndDerivatives=provide  SimscapeFilterOrder=2  InputFilterTimeConstant=0.001  UdotUserProvided=0
      settings: SourceProductBaseCode=PW,SS
  Simulink-PS Converter5 : nesl_utility/Simulink-PS Converter  PhysicalDomain=network_engine_domain  SubClassName=ps_input  LeftPortType=input  RightPortType=output  PseudoPeriodic=off  Frequencies=[]  NoiseDistribution=none  NoiseParameters=[]  Unit=1  AffineConversion=off  FilteringAndDerivatives=provide  SimscapeFilterOrder=2  InputFilterTimeConstant=0.001  UdotUserProvided=0
      settings: SourceProductBaseCode=PW,SS
  Solver Configuration : nesl_utility/Solver Configuration  PhysicalDomain=network_engine_domain  SubClassName=solver  LeftPortType=input  RightPortType=generic  Tones=[]  Harmonics=[]  SimulateNoise=off  Profile=off  UseLocalSampling=off  EnableSwitchedLinearOptims=on  FrequencyDomain=off  UseCCode=off  RelTol=0.001  AbsTol=1e-06  MinStep=1e-09  ToWorkspace=off  RevertToSquareIcSolve=off  NumHomotopyIterations=100  PhasorMode=off  PhasorModeNumHarmonics=1  DoDC=off  ResidualTolerance=1e-09  UseLocalSolver=off  LocalSolverChoice=NE_BACKWARD_EULER_ADVANCER  LocalSolverSampleTime=0.001  DoFixedCost=off  MaxNonlinIter=3  MaxModeIter=2  ComputeImpulses=off  ImpulseIterations=2  LinearAlgebra=auto  EquationFormulation=NE_TIME_EF  DelaysMemoryBudget=1024  AutomaticFiltering=on  FilteringTimeConstant=0.001  PartitionStorageMethod=AS_NEEDED  PartitionMemoryBudget=1024  PartitionMethod=ROBUST
      settings: SourceProductBaseCode=PW,SS
  Transform : sm_lib/Frames and Transforms/Rigid Transform  TranslationMethod=Cartesian  TranslationStandardOffset=0  TranslationLengthUnit=mm  TranslationStandardAxis=+Z  TranslationCartesianOffset=smiData.RigidTransform(13).translation  TranslationROffset=0  TranslationROffsetUnits=m  TranslationZOffset=0  TranslationZOffsetUnits=m  TranslationThetaOffset=0  TranslationThetaOffsetUnits=deg  RotationMethod=ArbitraryAxis  RotationAngleUnits=rad  RotationStandardAxis=+Z  RotationAngle=smiData.RigidTransform(13).angle  RotationArbitraryAxis=smiData.RigidTransform(13).axis  FollAlignAxisA=+X  BaseAlignAxisA=+Y  FollAlignAxisB=+Y  BaseAlignAxisB=+Z  RotationSequenceAxes=FollowerAxes  RotationSequence=XYX  RotationSequenceAngles=[0 0 0]  RotationSequenceAnglesUnits=deg  RotationMatrix=[1 0 0; 0 1 0; 0 0 1]
  World : sm_lib/Frames and Transforms/World Frame
  wires:
  psi/1 -> Simulink-PS Converter/1
  theta/1 -> Simulink-PS Converter1/1
  Constant1/1 -> Simulink-PS Converter2/1
  Constant2/1 -> Simulink-PS Converter3/1
  Gain/1 -> Simulink-PS Converter5/1
  Gain1/1 -> Simulink-PS Converter4/1
  thruster_2/1 -> Gain/1
  thruster_1/1 -> Gain1/1
  connections:
  AERO_Fork1_RIGID/RConn1 -- Rotational2/LConn1
  MechanismConfiguration/RConn1 -- Transform/LConn1 -- World/RConn1 -- Solver Configuration/RConn1
  AERO_Propeller1_RIGID/LConn1 -- Rotational5/RConn1
  AERO_Fork1_RIGID/LConn1 -- Rotational1/RConn1
  AERO_Propeller_Housing2_RIGID/LConn1 -- Rotational4/RConn1
  AERO_Arm1_RIGID/RConn2 -- Rotational3/LConn1
  AERO_Propeller_Housing2_RIGID/RConn1 -- Rotational6/LConn1
  AERO_Propeller_Housing1_RIGID/LConn1 -- Rotational3/RConn1
  AERO_Arm1_RIGID/RConn1 -- Rotational4/LConn1
  AERO_Propeller2_RIGID/LConn1 -- Rotational6/RConn1
  Transform/RConn1 -- AERO_Base1_RIGID/LConn1
  AERO_Arm1_RIGID/LConn1 -- Rotational2/RConn1
  AERO_Propeller_Housing1_RIGID/RConn1 -- Rotational5/LConn1
  AERO_Base1_RIGID/RConn1 -- Rotational1/LConn1
  Simulink-PS Converter/RConn1 -- Rotational1/LConn2
  Simulink-PS Converter1/RConn1 -- Rotational2/LConn2
  Simulink-PS Converter2/RConn1 -- Rotational4/LConn2
  Simulink-PS Converter3/RConn1 -- Rotational3/LConn2
  Simulink-PS Converter4/RConn1 -- Rotational5/LConn2
  Simulink-PS Converter5/RConn1 -- Rotational6/LConn2

== system Quanser_AERO_Simulation_2020b/Quanser AERO/Input Noise ==
  u : Inport
  Demux : Demux  Outputs=2
  Motor 0 Noise : simulink/Sources/Band-Limited White Noise  Cov=[noise.motor_0*ts]  Ts=ts  seed=[23341]
  Motor 1 Noise : simulink/Sources/Band-Limited White Noise  Cov=[noise.motor_1*ts]  Ts=ts  seed=[23341]
  Mux : Mux  Inputs=2
  Sum : Sum  Inputs=|++
  Sum1 : Sum  Inputs=++|
  u_noise : Outport  VectorParamsAs1DForOutWhenUnconnected=off
  wires:
  u/1 -> Demux/1
  Demux/2 -> Sum/1
  Demux/1 -> Sum1/2
  Motor 0 Noise/1 -> Sum1/1
  Motor 1 Noise/1 -> Sum/2
  Mux/1 -> u_noise/1
  Sum1/1 -> Mux/1
  Sum/1 -> Mux/2

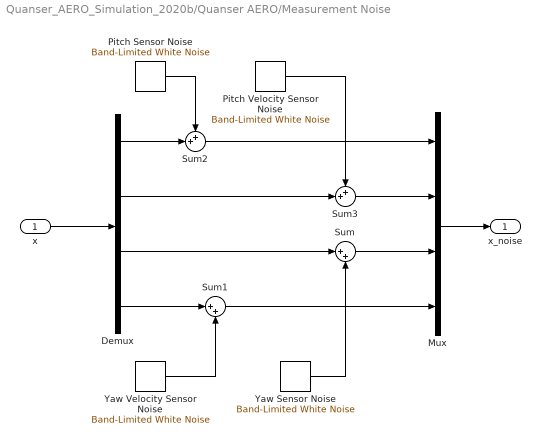
== system Quanser_AERO_Simulation_2020b/Quanser AERO/Measurement Noise ==
  x : Inport
  Demux : Demux
  Mux : Mux
  Pitch Sensor Noise : simulink/Sources/Band-Limited White Noise  Cov=[noise.pitch*ts]  Ts=ts  seed=[23341]
  Pitch Velocity Sensor Noise : simulink/Sources/Band-Limited White Noise  Cov=[noise.pitch_vel*ts]  Ts=ts  seed=[23341]
  Sum : Sum  Inputs=|++
  Sum1 : Sum  Inputs=|++
  Sum2 : Sum  Inputs=++|
  Sum3 : Sum  Inputs=++|
  Yaw Sensor Noise : simulink/Sources/Band-Limited White Noise  Cov=[noise.yaw*ts]  Ts=ts  seed=[23341]
  Yaw Velocity Sensor Noise : simulink/Sources/Band-Limited White Noise  Cov=[noise.yaw_vel*ts]  Ts=ts  seed=[23341]
  x_noise : Outport  VectorParamsAs1DForOutWhenUnconnected=off
  wires:
  x/1 -> Demux/1
  Demux/3 -> Sum/1
  Demux/4 -> Sum1/1
  Demux/1 -> Sum2/2
  Pitch Sensor Noise/1 -> Sum2/1
  Demux/2 -> Sum3/2
  Pitch Velocity Sensor Noise/1 -> Sum3/1
  Mux/1 -> x_noise/1
  Sum/1 -> Mux/3
  Sum3/1 -> Mux/2
  Sum2/1 -> Mux/1
  Sum1/1 -> Mux/4
  Yaw Sensor Noise/1 -> Sum/2
  Yaw Velocity Sensor Noise/1 -> Sum1/2

== system Quanser_AERO_Simulation_2020b/Quanser AERO/Quanser AERO System Dynamics ==
  x : Inport  OutDataTypeStr=double  PortDimensions=4  SampleTime=0
  u : Inport  Port=2  OutDataTypeStr=double  PortDimensions=2
  model : Inport  Port=3  OutDataTypeStr=double  PortDimensions=1
  MATLAB Function : MATLAB Function  TreatAsAtomicUnit=on
  Saturation : Saturate  UpperLimit=u_lim  LowerLimit=-u_lim
  x_dot : Outport  OutDataTypeStr=double  PortDimensions=4  SampleTime=0  VectorParamsAs1DForOutWhenUnconnected=off
  wires:
  u/1 -> Saturation/1
  MATLAB Function/1(x_dot) -> x_dot/1  "x_dot"
  x/1 -> MATLAB Function/1(x)
  model/1 -> MATLAB Function/3(model)
  Saturation/1 -> MATLAB Function/2(u)

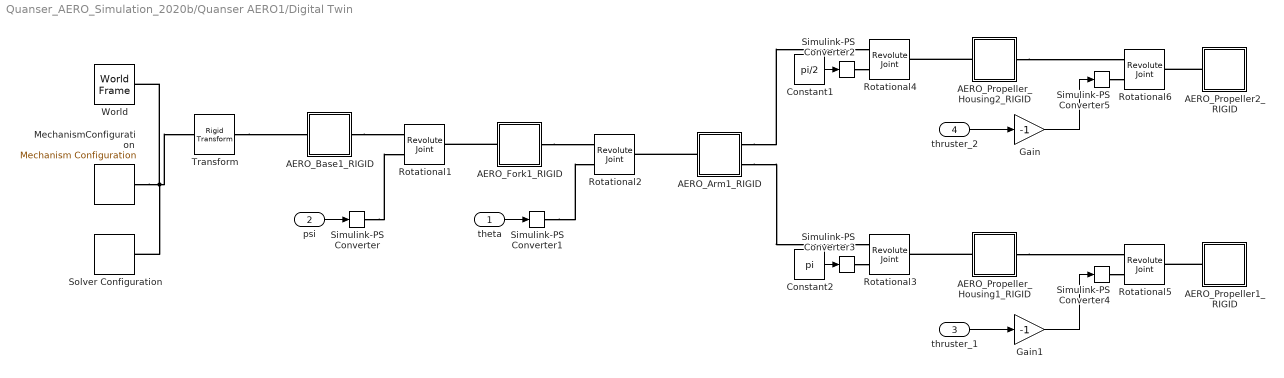
== system Quanser_AERO_Simulation_2020b/Quanser AERO1/Digital Twin ==
  theta : Inport
  psi : Inport  Port=2
  thruster_1 : Inport  Port=3
  thruster_2 : Inport  Port=4
  AERO_Arm1_RIGID : Subsystem
  AERO_Base1_RIGID : Subsystem
  AERO_Fork1_RIGID : Subsystem
  AERO_Propeller1_RIGID : Subsystem
  AERO_Propeller2_RIGID : Subsystem
  AERO_Propeller_Housing1_RIGID : Subsystem
  AERO_Propeller_Housing2_RIGID : Subsystem
  Constant1 : Constant  Value=pi/2
  Constant2 : Constant  Value=pi
  Gain : Gain  Gain=-1
  Gain1 : Gain  Gain=-1
  MechanismConfiguration : sm_lib/Utilities/Mechanism Configuration  UniformGravity=Constant  GravityVector=[0 -9.80665 0]  GravityVectorUnits=m/s^2  GravityUnits=m/s^2  LinearizationDelta=0.001  JointModeTransitionNonlinearIterations=2
  Rotational1 : sm_lib/Joints/Revolute Joint  JointMode=Normal  SenseConstraintForce=off  SenseConstraintForceX=off  SenseConstraintForceY=off  SenseConstraintForceZ=off  SenseConstraintTorque=off  SenseConstraintTorqueX=off  SenseConstraintTorqueY=off  SenseConstraintTorqueZ=off  SenseTotalForce=off  SenseTotalForceX=off  SenseTotalForceY=off  SenseTotalForceZ=off  SenseTotalTorque=off  SenseTotalTorqueX=off  SenseTotalTorqueY=off  SenseTotalTorqueZ=off  CompositeWrenchDir=FollowerOnBase  CompositeWrenchFrame=BaseFrame  EquilibriumPosition=0  EquilibriumPositionUnits=deg  SpringStiffness=0  SpringStiffnessUnits=N*m/deg  DampingCoefficient=0  DampingCoefficientUnits=N*m/(deg/s)  TorqueActuationMode=ComputedTorque  MotionActuationMode=InputMotion  SensePosition=off  SenseVelocity=off  SenseAcceleration=off  SenseTorqueForce=off  SenseLowerLimitTorqueForce=off  SenseUpperLimitTorqueForce=off  LowerLimitSpecify=off  LowerLimitBound=-90  LowerLimitBoundUnits=deg  LowerLimitStiffness=1e4  LowerLimitStiffnessUnits=N*m/deg  LowerLimitDamping=10  LowerLimitDampingUnits=N*m/(deg/s)  LowerLimitTransitionRegionWidth=0.1  LowerLimitTransitionRegionWidthUnits=deg  UpperLimitSpecify=off  UpperLimitBound=90  UpperLimitBoundUnits=deg  UpperLimitStiffness=1e4  UpperLimitStiffnessUnits=N*m/deg  UpperLimitDamping=10  UpperLimitDampingUnits=N*m/(deg/s)  UpperLimitTransitionRegionWidth=0.1  UpperLimitTransitionRegionWidthUnits=deg  PositionTargetSpecify=on  PositionTargetPriority=Low  PositionTargetValue=smiData.RevoluteJoint(4).Rz.Pos  PositionTargetValueUnits=deg  VelocityTargetSpecify=off  VelocityTargetPriority=High  VelocityTargetValue=0  VelocityTargetValueUnits=deg/s
  Rotational2 : sm_lib/Joints/Revolute Joint  JointMode=Normal  SenseConstraintForce=off  SenseConstraintForceX=off  SenseConstraintForceY=off  SenseConstraintForceZ=off  SenseConstraintTorque=off  SenseConstraintTorqueX=off  SenseConstraintTorqueY=off  SenseConstraintTorqueZ=off  SenseTotalForce=off  SenseTotalForceX=off  SenseTotalForceY=off  SenseTotalForceZ=off  SenseTotalTorque=off  SenseTotalTorqueX=off  SenseTotalTorqueY=off  SenseTotalTorqueZ=off  CompositeWrenchDir=FollowerOnBase  CompositeWrenchFrame=BaseFrame  EquilibriumPosition=0  EquilibriumPositionUnits=deg  SpringStiffness=0  SpringStiffnessUnits=N*m/deg  DampingCoefficient=0  DampingCoefficientUnits=N*m/(deg/s)  TorqueActuationMode=ComputedTorque  MotionActuationMode=InputMotion  SensePosition=off  SenseVelocity=off  SenseAcceleration=off  SenseTorqueForce=off  SenseLowerLimitTorqueForce=off  SenseUpperLimitTorqueForce=off  LowerLimitSpecify=off  LowerLimitBound=-90  LowerLimitBoundUnits=deg  LowerLimitStiffness=1e4  LowerLimitStiffnessUnits=N*m/deg  LowerLimitDamping=10  LowerLimitDampingUnits=N*m/(deg/s)  LowerLimitTransitionRegionWidth=0.1  LowerLimitTransitionRegionWidthUnits=deg  UpperLimitSpecify=off  UpperLimitBound=90  UpperLimitBoundUnits=deg  UpperLimitStiffness=1e4  UpperLimitStiffnessUnits=N*m/deg  UpperLimitDamping=10  UpperLimitDampingUnits=N*m/(deg/s)  UpperLimitTransitionRegionWidth=0.1  UpperLimitTransitionRegionWidthUnits=deg  PositionTargetSpecify=on  PositionTargetPriority=Low  PositionTargetValue=smiData.RevoluteJoint(1).Rz.Pos  PositionTargetValueUnits=deg  VelocityTargetSpecify=off  VelocityTargetPriority=High  VelocityTargetValue=0  VelocityTargetValueUnits=deg/s
  Rotational3 : sm_lib/Joints/Revolute Joint  JointMode=Normal  SenseConstraintForce=off  SenseConstraintForceX=off  SenseConstraintForceY=off  SenseConstraintForceZ=off  SenseConstraintTorque=off  SenseConstraintTorqueX=off  SenseConstraintTorqueY=off  SenseConstraintTorqueZ=off  SenseTotalForce=off  SenseTotalForceX=off  SenseTotalForceY=off  SenseTotalForceZ=off  SenseTotalTorque=off  SenseTotalTorqueX=off  SenseTotalTorqueY=off  SenseTotalTorqueZ=off  CompositeWrenchDir=FollowerOnBase  CompositeWrenchFrame=BaseFrame  EquilibriumPosition=0  EquilibriumPositionUnits=deg  SpringStiffness=0  SpringStiffnessUnits=N*m/deg  DampingCoefficient=0  DampingCoefficientUnits=N*m/(deg/s)  TorqueActuationMode=ComputedTorque  MotionActuationMode=InputMotion  SensePosition=off  SenseVelocity=off  SenseAcceleration=off  SenseTorqueForce=off  SenseLowerLimitTorqueForce=off  SenseUpperLimitTorqueForce=off  LowerLimitSpecify=off  LowerLimitBound=-90  LowerLimitBoundUnits=deg  LowerLimitStiffness=1e4  LowerLimitStiffnessUnits=N*m/deg  LowerLimitDamping=10  LowerLimitDampingUnits=N*m/(deg/s)  LowerLimitTransitionRegionWidth=0.1  LowerLimitTransitionRegionWidthUnits=deg  UpperLimitSpecify=off  UpperLimitBound=90  UpperLimitBoundUnits=deg  UpperLimitStiffness=1e4  UpperLimitStiffnessUnits=N*m/deg  UpperLimitDamping=10  UpperLimitDampingUnits=N*m/(deg/s)  UpperLimitTransitionRegionWidth=0.1  UpperLimitTransitionRegionWidthUnits=deg  PositionTargetSpecify=on  PositionTargetPriority=High  PositionTargetValue=smiData.RevoluteJoint(2).Rz.Pos  PositionTargetValueUnits=deg  VelocityTargetSpecify=off  VelocityTargetPriority=High  VelocityTargetValue=0  VelocityTargetValueUnits=deg/s
  Rotational4 : sm_lib/Joints/Revolute Joint  JointMode=Normal  SenseConstraintForce=off  SenseConstraintForceX=off  SenseConstraintForceY=off  SenseConstraintForceZ=off  SenseConstraintTorque=off  SenseConstraintTorqueX=off  SenseConstraintTorqueY=off  SenseConstraintTorqueZ=off  SenseTotalForce=off  SenseTotalForceX=off  SenseTotalForceY=off  SenseTotalForceZ=off  SenseTotalTorque=off  SenseTotalTorqueX=off  SenseTotalTorqueY=off  SenseTotalTorqueZ=off  CompositeWrenchDir=FollowerOnBase  CompositeWrenchFrame=BaseFrame  EquilibriumPosition=0  EquilibriumPositionUnits=deg  SpringStiffness=0  SpringStiffnessUnits=N*m/deg  DampingCoefficient=0  DampingCoefficientUnits=N*m/(deg/s)  TorqueActuationMode=ComputedTorque  MotionActuationMode=InputMotion  SensePosition=off  SenseVelocity=off  SenseAcceleration=off  SenseTorqueForce=off  SenseLowerLimitTorqueForce=off  SenseUpperLimitTorqueForce=off  LowerLimitSpecify=off  LowerLimitBound=-90  LowerLimitBoundUnits=deg  LowerLimitStiffness=1e4  LowerLimitStiffnessUnits=N*m/deg  LowerLimitDamping=10  LowerLimitDampingUnits=N*m/(deg/s)  LowerLimitTransitionRegionWidth=0.1  LowerLimitTransitionRegionWidthUnits=deg  UpperLimitSpecify=off  UpperLimitBound=90  UpperLimitBoundUnits=deg  UpperLimitStiffness=1e4  UpperLimitStiffnessUnits=N*m/deg  UpperLimitDamping=10  UpperLimitDampingUnits=N*m/(deg/s)  UpperLimitTransitionRegionWidth=0.1  UpperLimitTransitionRegionWidthUnits=deg  PositionTargetSpecify=on  PositionTargetPriority=Low  PositionTargetValue=smiData.RevoluteJoint(3).Rz.Pos  PositionTargetValueUnits=deg  VelocityTargetSpecify=off  VelocityTargetPriority=High  VelocityTargetValue=0  VelocityTargetValueUnits=deg/s
  Rotational5 : sm_lib/Joints/Revolute Joint  JointMode=Normal  SenseConstraintForce=off  SenseConstraintForceX=off  SenseConstraintForceY=off  SenseConstraintForceZ=off  SenseConstraintTorque=off  SenseConstraintTorqueX=off  SenseConstraintTorqueY=off  SenseConstraintTorqueZ=off  SenseTotalForce=off  SenseTotalForceX=off  SenseTotalForceY=off  SenseTotalForceZ=off  SenseTotalTorque=off  SenseTotalTorqueX=off  SenseTotalTorqueY=off  SenseTotalTorqueZ=off  CompositeWrenchDir=FollowerOnBase  CompositeWrenchFrame=BaseFrame  EquilibriumPosition=0  EquilibriumPositionUnits=deg  SpringStiffness=0  SpringStiffnessUnits=N*m/deg  DampingCoefficient=0.000001  DampingCoefficientUnits=N*m/(deg/s)  TorqueActuationMode=InputTorque  MotionActuationMode=ComputedMotion  SensePosition=off  SenseVelocity=off  SenseAcceleration=off  SenseTorqueForce=off  SenseLowerLimitTorqueForce=off  SenseUpperLimitTorqueForce=off  LowerLimitSpecify=off  LowerLimitBound=-90  LowerLimitBoundUnits=deg  LowerLimitStiffness=1e4  LowerLimitStiffnessUnits=N*m/deg  LowerLimitDamping=10  LowerLimitDampingUnits=N*m/(deg/s)  LowerLimitTransitionRegionWidth=0.1  LowerLimitTransitionRegionWidthUnits=deg  UpperLimitSpecify=off  UpperLimitBound=90  UpperLimitBoundUnits=deg  UpperLimitStiffness=1e4  UpperLimitStiffnessUnits=N*m/deg  UpperLimitDamping=10  UpperLimitDampingUnits=N*m/(deg/s)  UpperLimitTransitionRegionWidth=0.1  UpperLimitTransitionRegionWidthUnits=deg  PositionTargetSpecify=on  PositionTargetPriority=Low  PositionTargetValue=smiData.RevoluteJoint(5).Rz.Pos  PositionTargetValueUnits=deg  VelocityTargetSpecify=off  VelocityTargetPriority=High  VelocityTargetValue=0  VelocityTargetValueUnits=deg/s
  Rotational6 : sm_lib/Joints/Revolute Joint  JointMode=Normal  SenseConstraintForce=off  SenseConstraintForceX=off  SenseConstraintForceY=off  SenseConstraintForceZ=off  SenseConstraintTorque=off  SenseConstraintTorqueX=off  SenseConstraintTorqueY=off  SenseConstraintTorqueZ=off  SenseTotalForce=off  SenseTotalForceX=off  SenseTotalForceY=off  SenseTotalForceZ=off  SenseTotalTorque=off  SenseTotalTorqueX=off  SenseTotalTorqueY=off  SenseTotalTorqueZ=off  CompositeWrenchDir=FollowerOnBase  CompositeWrenchFrame=BaseFrame  EquilibriumPosition=0  EquilibriumPositionUnits=deg  SpringStiffness=0  SpringStiffnessUnits=N*m/deg  DampingCoefficient=0.000001  DampingCoefficientUnits=N*m/(rad/s)  TorqueActuationMode=InputTorque  MotionActuationMode=ComputedMotion  SensePosition=off  SenseVelocity=off  SenseAcceleration=off  SenseTorqueForce=off  SenseLowerLimitTorqueForce=off  SenseUpperLimitTorqueForce=off  LowerLimitSpecify=off  LowerLimitBound=-90  LowerLimitBoundUnits=deg  LowerLimitStiffness=1e4  LowerLimitStiffnessUnits=N*m/deg  LowerLimitDamping=10  LowerLimitDampingUnits=N*m/(deg/s)  LowerLimitTransitionRegionWidth=0.1  LowerLimitTransitionRegionWidthUnits=deg  UpperLimitSpecify=off  UpperLimitBound=90  UpperLimitBoundUnits=deg  UpperLimitStiffness=1e4  UpperLimitStiffnessUnits=N*m/deg  UpperLimitDamping=10  UpperLimitDampingUnits=N*m/(deg/s)  UpperLimitTransitionRegionWidth=0.1  UpperLimitTransitionRegionWidthUnits=deg  PositionTargetSpecify=on  PositionTargetPriority=Low  PositionTargetValue=smiData.RevoluteJoint(6).Rz.Pos  PositionTargetValueUnits=deg  VelocityTargetSpecify=off  VelocityTargetPriority=High  VelocityTargetValue=0  VelocityTargetValueUnits=deg/s
  Simulink-PS Converter{,1..3} (4 alike) : nesl_utility/Simulink-PS Converter  PhysicalDomain=network_engine_domain  SubClassName=ps_input  LeftPortType=input  RightPortType=output  PseudoPeriodic=off  Frequencies=[]  NoiseDistribution=none  NoiseParameters=[]  Unit=1  AffineConversion=off  FilteringAndDerivatives=filter  SimscapeFilterOrder=2  InputFilterTimeConstant=0.001  UdotUserProvided=0
      settings: SourceProductBaseCode=PW,SS
  Simulink-PS Converter4 : nesl_utility/Simulink-PS Converter  PhysicalDomain=network_engine_domain  SubClassName=ps_input  LeftPortType=input  RightPortType=output  PseudoPeriodic=off  Frequencies=[]  NoiseDistribution=none  NoiseParameters=[]  Unit=1  AffineConversion=off  FilteringAndDerivatives=provide  SimscapeFilterOrder=2  InputFilterTimeConstant=0.001  UdotUserProvided=0
      settings: SourceProductBaseCode=PW,SS
  Simulink-PS Converter5 : nesl_utility/Simulink-PS Converter  PhysicalDomain=network_engine_domain  SubClassName=ps_input  LeftPortType=input  RightPortType=output  PseudoPeriodic=off  Frequencies=[]  NoiseDistribution=none  NoiseParameters=[]  Unit=1  AffineConversion=off  FilteringAndDerivatives=provide  SimscapeFilterOrder=2  InputFilterTimeConstant=0.001  UdotUserProvided=0
      settings: SourceProductBaseCode=PW,SS
  Solver Configuration : nesl_utility/Solver Configuration  PhysicalDomain=network_engine_domain  SubClassName=solver  LeftPortType=input  RightPortType=generic  Tones=[]  Harmonics=[]  SimulateNoise=off  Profile=off  UseLocalSampling=off  EnableSwitchedLinearOptims=on  FrequencyDomain=off  UseCCode=off  RelTol=0.001  AbsTol=1e-06  MinStep=1e-09  ToWorkspace=off  RevertToSquareIcSolve=off  NumHomotopyIterations=100  PhasorMode=off  PhasorModeNumHarmonics=1  DoDC=off  ResidualTolerance=1e-09  UseLocalSolver=off  LocalSolverChoice=NE_BACKWARD_EULER_ADVANCER  LocalSolverSampleTime=0.001  DoFixedCost=off  MaxNonlinIter=3  MaxModeIter=2  ComputeImpulses=off  ImpulseIterations=2  LinearAlgebra=auto  EquationFormulation=NE_TIME_EF  DelaysMemoryBudget=1024  AutomaticFiltering=on  FilteringTimeConstant=0.001  PartitionStorageMethod=AS_NEEDED  PartitionMemoryBudget=1024  PartitionMethod=ROBUST
      settings: SourceProductBaseCode=PW,SS
  Transform : sm_lib/Frames and Transforms/Rigid Transform  TranslationMethod=Cartesian  TranslationStandardOffset=0  TranslationLengthUnit=mm  TranslationStandardAxis=+Z  TranslationCartesianOffset=smiData.RigidTransform(13).translation  TranslationROffset=0  TranslationROffsetUnits=m  TranslationZOffset=0  TranslationZOffsetUnits=m  TranslationThetaOffset=0  TranslationThetaOffsetUnits=deg  RotationMethod=ArbitraryAxis  RotationAngleUnits=rad  RotationStandardAxis=+Z  RotationAngle=smiData.RigidTransform(13).angle  RotationArbitraryAxis=smiData.RigidTransform(13).axis  FollAlignAxisA=+X  BaseAlignAxisA=+Y  FollAlignAxisB=+Y  BaseAlignAxisB=+Z  RotationSequenceAxes=FollowerAxes  RotationSequence=XYX  RotationSequenceAngles=[0 0 0]  RotationSequenceAnglesUnits=deg  RotationMatrix=[1 0 0; 0 1 0; 0 0 1]
  World : sm_lib/Frames and Transforms/World Frame
  wires:
  psi/1 -> Simulink-PS Converter/1
  theta/1 -> Simulink-PS Converter1/1
  Constant1/1 -> Simulink-PS Converter2/1
  Constant2/1 -> Simulink-PS Converter3/1
  Gain/1 -> Simulink-PS Converter5/1
  Gain1/1 -> Simulink-PS Converter4/1
  thruster_2/1 -> Gain/1
  thruster_1/1 -> Gain1/1
  connections:
  AERO_Fork1_RIGID/RConn1 -- Rotational2/LConn1
  MechanismConfiguration/RConn1 -- Transform/LConn1 -- World/RConn1 -- Solver Configuration/RConn1
  AERO_Propeller1_RIGID/LConn1 -- Rotational5/RConn1
  AERO_Fork1_RIGID/LConn1 -- Rotational1/RConn1
  AERO_Propeller_Housing2_RIGID/LConn1 -- Rotational4/RConn1
  AERO_Arm1_RIGID/RConn2 -- Rotational3/LConn1
  AERO_Propeller_Housing2_RIGID/RConn1 -- Rotational6/LConn1
  AERO_Propeller_Housing1_RIGID/LConn1 -- Rotational3/RConn1
  AERO_Arm1_RIGID/RConn1 -- Rotational4/LConn1
  AERO_Propeller2_RIGID/LConn1 -- Rotational6/RConn1
  Transform/RConn1 -- AERO_Base1_RIGID/LConn1
  AERO_Arm1_RIGID/LConn1 -- Rotational2/RConn1
  AERO_Propeller_Housing1_RIGID/RConn1 -- Rotational5/LConn1
  AERO_Base1_RIGID/RConn1 -- Rotational1/LConn1
  Simulink-PS Converter/RConn1 -- Rotational1/LConn2
  Simulink-PS Converter1/RConn1 -- Rotational2/LConn2
  Simulink-PS Converter2/RConn1 -- Rotational4/LConn2
  Simulink-PS Converter3/RConn1 -- Rotational3/LConn2
  Simulink-PS Converter4/RConn1 -- Rotational5/LConn2
  Simulink-PS Converter5/RConn1 -- Rotational6/LConn2

== system Quanser_AERO_Simulation_2020b/Quanser AERO1/Input Noise ==
  u : Inport
  Demux : Demux  Outputs=2
  Motor 0 Noise : simulink/Sources/Band-Limited White Noise  Cov=[noise.motor_0*ts]  Ts=ts  seed=[23341]
  Motor 1 Noise : simulink/Sources/Band-Limited White Noise  Cov=[noise.motor_1*ts]  Ts=ts  seed=[23341]
  Mux : Mux  Inputs=2
  Sum : Sum  Inputs=|++
  Sum1 : Sum  Inputs=++|
  u_noise : Outport  VectorParamsAs1DForOutWhenUnconnected=off
  wires:
  u/1 -> Demux/1
  Demux/2 -> Sum/1
  Demux/1 -> Sum1/2
  Motor 0 Noise/1 -> Sum1/1
  Motor 1 Noise/1 -> Sum/2
  Mux/1 -> u_noise/1
  Sum1/1 -> Mux/1
  Sum/1 -> Mux/2

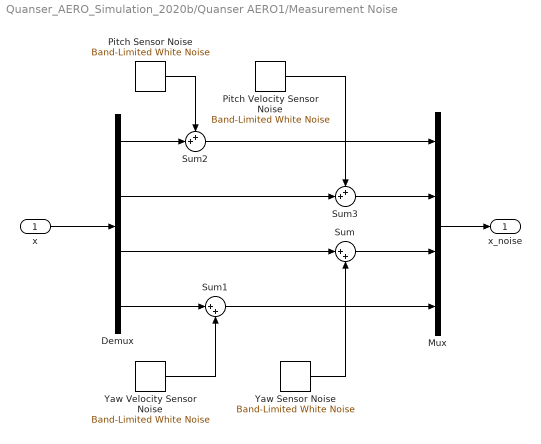
== system Quanser_AERO_Simulation_2020b/Quanser AERO1/Measurement Noise ==
  x : Inport
  Demux : Demux
  Mux : Mux
  Pitch Sensor Noise : simulink/Sources/Band-Limited White Noise  Cov=[noise.pitch*ts]  Ts=ts  seed=[23341]
  Pitch Velocity Sensor Noise : simulink/Sources/Band-Limited White Noise  Cov=[noise.pitch_vel*ts]  Ts=ts  seed=[23341]
  Sum : Sum  Inputs=|++
  Sum1 : Sum  Inputs=|++
  Sum2 : Sum  Inputs=++|
  Sum3 : Sum  Inputs=++|
  Yaw Sensor Noise : simulink/Sources/Band-Limited White Noise  Cov=[noise.yaw*ts]  Ts=ts  seed=[23341]
  Yaw Velocity Sensor Noise : simulink/Sources/Band-Limited White Noise  Cov=[noise.yaw_vel*ts]  Ts=ts  seed=[23341]
  x_noise : Outport  VectorParamsAs1DForOutWhenUnconnected=off
  wires:
  x/1 -> Demux/1
  Demux/3 -> Sum/1
  Demux/4 -> Sum1/1
  Demux/1 -> Sum2/2
  Pitch Sensor Noise/1 -> Sum2/1
  Demux/2 -> Sum3/2
  Pitch Velocity Sensor Noise/1 -> Sum3/1
  Mux/1 -> x_noise/1
  Sum/1 -> Mux/3
  Sum3/1 -> Mux/2
  Sum2/1 -> Mux/1
  Sum1/1 -> Mux/4
  Yaw Sensor Noise/1 -> Sum/2
  Yaw Velocity Sensor Noise/1 -> Sum1/2

== system Quanser_AERO_Simulation_2020b/Quanser AERO1/Quanser AERO System Dynamics ==
  x : Inport  OutDataTypeStr=double  PortDimensions=4  SampleTime=0
  u : Inport  Port=2  OutDataTypeStr=double  PortDimensions=2
  model : Inport  Port=3  OutDataTypeStr=double  PortDimensions=1
  MATLAB Function : MATLAB Function  TreatAsAtomicUnit=on
  Saturation : Saturate  UpperLimit=u_lim  LowerLimit=-u_lim
  x_dot : Outport  OutDataTypeStr=double  PortDimensions=4  SampleTime=0  VectorParamsAs1DForOutWhenUnconnected=off
  wires:
  u/1 -> Saturation/1
  MATLAB Function/1(x_dot) -> x_dot/1  "x_dot"
  x/1 -> MATLAB Function/1(x)
  model/1 -> MATLAB Function/3(model)
  Saturation/1 -> MATLAB Function/2(u)
